simulink model "torqueBalancing"  (Simulink 8.7)
settings: Solver=FixedStepDiscrete  StartTime=0.0  StopTime="CONFIG.SIMULATION_TIME "  FixedStep=CONFIG.Ts  RelTol=1e-3
InitFcn:
  | cd(fileparts(which(bdroot)));
  | initTorqueBalancing;
values from neighbouring files (symbols this model uses):
  baseToWorldRotationPort = ['/' WBT_modelName '/floatingBaseRotationMatrix:i']    [initTorqueBalancing.m]
  WBT_modelName = 'matlabTorqueBalancing'    [initTorqueBalancing.m]
undefined symbols (not defined in the file or in its folder): bVectorConstraints, CONFIG, ConstraintsMatrix, DiscIntNeverNeededParam, gain, references, reg, ROBOT_DOF, ROBOT_DOF_FOR_SIMULINK, sat, SM, sm, WBT_robotName
libraries: WBToolboxLibrary x119, simulink x11
(part 2 of 3)

== system torqueBalancing/DesValues/Internal coordinator/nu ==
  qj : Inport
  w_H_b : Inport  Port=2
  "constraints " : Inport  Port=3
  Get Estimate : WBToolboxLibrary/wholeBodyStates/Get Estimate  estimateType=Joints Velocity  robotName=WBT_robotName  localName=WBT_modelName  wbiFile=WBT_wbiFilename  wbiList=WBT_wbiList
  Jacobian l_sole : WBToolboxLibrary/wholeBodyModel/Jacobians/Jacobian  frameName='l_sole'  robotName=WBT_robotName  localName=WBT_modelName  wbiFile=WBT_wbiFilename  wbiList=WBT_wbiList
  Jacobian r_sole : WBToolboxLibrary/wholeBodyModel/Jacobians/Jacobian  frameName='r_sole'  robotName=WBT_robotName  localName=WBT_modelName  wbiFile=WBT_wbiFilename  wbiList=WBT_wbiList
  MATLAB Function : MATLAB Function  TreatAsAtomicUnit=on
  Mux : Mux  Inputs=2
  vb + Dqj : Outport
  wires:
  Get Estimate/1 -> MATLAB Function/4(qD), Mux/2
  Mux/1 -> vb + Dqj/1
  Jacobian r_sole/1 -> MATLAB Function/2(JcRightFoot)
  "constraints "/1 -> MATLAB Function/3(activeFeetConstraints)
  MATLAB Function/1(y) -> Mux/1
  Jacobian l_sole/1 -> MATLAB Function/1(JcLeftFoot)
  qj/1 -> Jacobian r_sole/2, Jacobian l_sole/2
  w_H_b/1 -> Jacobian r_sole/1, Jacobian l_sole/1

== system torqueBalancing/DesValues/Internal coordinator/refGen ==
  xCom(0) : Inport
  qj(0) : Inport  Port=2
  Enable : EnablePort
  Clock1 : Clock
  refGenFCN : MATLAB Function  TreatAsAtomicUnit=on
  qDes : Outport
  CoMrefs : Outport  Port=2
  wires:
  refGenFCN/2(desired_x_dx_ddx_CoM) -> CoMrefs/1
  xCom(0)/1 -> refGenFCN/1(xCom0)
  Clock1/1 -> refGenFCN/3(t)
  qj(0)/1 -> refGenFCN/2(q0)
  refGenFCN/1(qDes) -> qDes/1

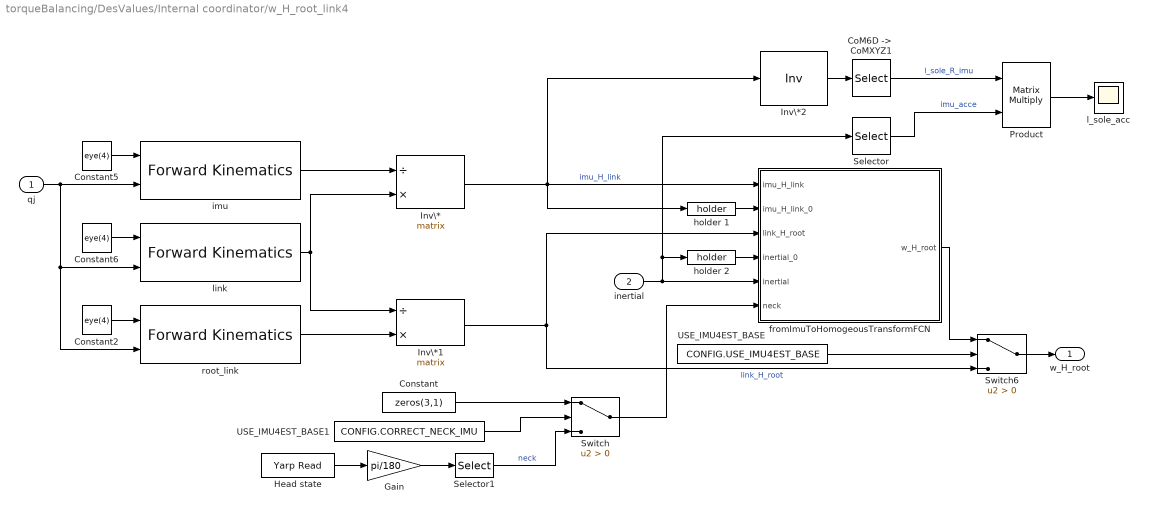
== system torqueBalancing/DesValues/Internal coordinator/w_H_root_link4 ==
  qj : Inport
  inertial : Inport  Port=2
  "CoM6D ->  CoMXYZ1" : Selector  NumberOfDimensions=2  InputPortWidth=7  IndexOptions=Index vector (dialog),Index vector (dialog)  Indices=[1 2 3],[1 2 3]  OutputSizes=1,1
  Constant : Constant  Value=zeros(3,1)
  Constant2 : Constant  Value=eye(4)
  Constant5 : Constant  Value=eye(4)
  Constant6 : Constant  Value=eye(4)
  Gain : Gain  Gain=pi/180
  Head state : WBToolboxLibrary/Utilities/Yarp Read  portName=[WBT_robotName, '/head/state:o']  signalSize=6  blocking=off  timestamp=off  autoconnect=on  errorOnConnection=off
  Inv\* : Product  Inputs=/*  Multiplication=Matrix(*)
  Inv\*1 : Product  Inputs=/*  Multiplication=Matrix(*)
  Inv\*2 : Product  Inputs=/  Multiplication=Matrix(*)
  Product : Product  Multiplication=Matrix(*)
  Selector : Selector  InputPortWidth=12  IndexOptions=Index vector (dialog)  Indices=[4 5 6 ]  OutputSizes=1
  Selector1 : Selector  InputPortWidth=6  IndexOptions=Index vector (dialog)  Indices=[1:3]  OutputSizes=1
  Switch : Switch  Criteria=u2 > Threshold
  Switch6 : Switch  Criteria=u2 > Threshold
  USE_IMU4EST_BASE : Constant  Value=CONFIG.USE_IMU4EST_BASE
  USE_IMU4EST_BASE1 : Constant  Value=CONFIG.CORRECT_NECK_IMU
  fromImuToHomogeousTransformFCN : MATLAB Function  TreatAsAtomicUnit=on
  holder 1 : WBToolboxLibrary/Utilities/holder 
  holder 2 : WBToolboxLibrary/Utilities/holder 
  imu : WBToolboxLibrary/wholeBodyModel/Kinematics/Forward Kinematics  frameName=imu_link_name  robotName=WBT_robotName  localName=WBT_modelName  wbiFile=WBT_wbiFilename  wbiList=WBT_wbiList
  l_sole_acc : Scope
  link : WBToolboxLibrary/wholeBodyModel/Kinematics/Forward Kinematics  frameName=link_name  robotName=WBT_robotName  localName=WBT_modelName  wbiFile=WBT_wbiFilename  wbiList=WBT_wbiList
  root_link : WBToolboxLibrary/wholeBodyModel/Kinematics/Forward Kinematics  frameName=root_link_name  robotName=WBT_robotName  localName=WBT_modelName  wbiFile=WBT_wbiFilename  wbiList=WBT_wbiList
  w_H_root : Outport
  wires:
  Constant5/1 -> imu/1
  Inv\*/1 -> Inv\*2/1, holder 1/1, fromImuToHomogeousTransformFCN/1(imu_H_link)  "imu_H_link"
  imu/1 -> Inv\*/1
  Constant6/1 -> link/1
  Inv\*1/1 -> Switch6/3, fromImuToHomogeousTransformFCN/3(link_H_root)  "link_H_root"
  link/1 -> Inv\*/2, Inv\*1/1
  inertial/1 -> Selector/1, holder 2/1, fromImuToHomogeousTransformFCN/5(inertial)
  Switch6/1 -> w_H_root/1
  USE_IMU4EST_BASE/1 -> Switch6/2
  fromImuToHomogeousTransformFCN/1(w_H_root) -> Switch6/1
  Constant2/1 -> root_link/1
  qj/1 -> root_link/2, link/2, imu/2
  root_link/1 -> Inv\*1/2
  holder 1/1 -> fromImuToHomogeousTransformFCN/2(imu_H_link_0)
  holder 2/1 -> fromImuToHomogeousTransformFCN/4(inertial_0)
  Inv\*2/1 -> "CoM6D ->  CoMXYZ1"/1
  "CoM6D ->  CoMXYZ1"/1 -> Product/1  "l_sole_R_imu"
  Selector/1 -> Product/2  "imu_acce"
  Product/1 -> l_sole_acc/1
  Head state/1 -> Gain/1
  Selector1/1 -> Switch/3  "neck"
  Constant/1 -> Switch/1
  USE_IMU4EST_BASE1/1 -> Switch/2
  Switch/1 -> fromImuToHomogeousTransformFCN/6(neck)
  Gain/1 -> Selector1/1

== system torqueBalancing/DesValues/Internal coordinator/xCom ==
  w_H_b : Inport
  qj : Inport  Port=2
  "CoM6D ->  CoMXYZ2" : Selector  NumberOfDimensions=2  InputPortWidth=7  IndexOptions=Index vector (dialog),Index vector (dialog)  Indices=[1 2 3],[4]  OutputSizes=1,1
  com : WBToolboxLibrary/wholeBodyModel/Kinematics/Forward Kinematics  frameName='com'  robotName=WBT_robotName  localName=WBT_modelName  wbiFile=WBT_wbiFilename  wbiList=WBT_wbiList
  xCom : Outport
  wires:
  qj/1 -> com/2
  "CoM6D ->  CoMXYZ2"/1 -> xCom/1
  com/1 -> "CoM6D ->  CoMXYZ2"/1
  w_H_b/1 -> com/1

== system torqueBalancing/DesValues/State Machine/Visualise extrnal wrenches   ==
  wL_WBDT : Inport
  wR_WBDT : Inport  Port=2
  Enable : EnablePort
  Constant : Constant  Value=sm.wrench.thresholdContactOn
  Constant2 : Constant  Value=sm.wrench.thresholdContactOff
  left foot ext wrench : Scope  NumInputPorts=3
  right foot ext wrench : Scope  NumInputPorts=3
  wires:
  Constant/1 -> left foot ext wrench/2, right foot ext wrench/2  "thresholdContactOn"
  wR_WBDT/1 -> right foot ext wrench/1  "wR_WBDT"
  wL_WBDT/1 -> left foot ext wrench/1  "wL_WBDT"
  Constant2/1 -> left foot ext wrench/3, right foot ext wrench/3  "thresholdContactOff"

== system torqueBalancing/DesValues/State Machine/nu ==
  qj : Inport
  w_H_b : Inport  Port=2
  "constraints " : Inport  Port=3
  Get Estimate : WBToolboxLibrary/wholeBodyStates/Get Estimate  estimateType=Joints Velocity  robotName=WBT_robotName  localName=WBT_modelName  wbiFile=WBT_wbiFilename  wbiList=WBT_wbiList
  Jacobian l_sole : WBToolboxLibrary/wholeBodyModel/Jacobians/Jacobian  frameName='l_sole'  robotName=WBT_robotName  localName=WBT_modelName  wbiFile=WBT_wbiFilename  wbiList=WBT_wbiList
  Jacobian r_sole : WBToolboxLibrary/wholeBodyModel/Jacobians/Jacobian  frameName='r_sole'  robotName=WBT_robotName  localName=WBT_modelName  wbiFile=WBT_wbiFilename  wbiList=WBT_wbiList
  MATLAB Function : MATLAB Function  TreatAsAtomicUnit=on
  Mux : Mux  Inputs=2
  vb + Dqj : Outport
  wires:
  Get Estimate/1 -> MATLAB Function/4(qD), Mux/2
  Mux/1 -> vb + Dqj/1
  Jacobian r_sole/1 -> MATLAB Function/2(JcRightFoot)
  "constraints "/1 -> MATLAB Function/3(activeFeetConstraints)
  MATLAB Function/1(y) -> Mux/1
  Jacobian l_sole/1 -> MATLAB Function/1(JcLeftFoot)
  qj/1 -> Jacobian r_sole/2, Jacobian l_sole/2
  w_H_b/1 -> Jacobian r_sole/1, Jacobian l_sole/1

== system torqueBalancing/DesValues/State Machine/visualise inertial ==
  jointAngles : Inport
  inertial : Inport  Port=2
  Enable : EnablePort
  Inv\* : Product  Inputs=/*  Multiplication=Matrix(*)
  Inv\*1 : Product  Inputs=/*  Multiplication=Matrix(*)
  Visualize hom transf1 : Subsystem
  Visualize hom transf2 : Subsystem
  Visualize hom transf3 : Subsystem
  Visualize hom transf4 : Subsystem
  Visualize hom transf5 : Subsystem
  Visualize hom transf6 : Subsystem
  "inertial -> rpy" : Selector  InputPortWidth=12  IndexOptions=Index vector (dialog)  Indices=[1 2 3]  OutputSizes=1
  l_sole_H_root_link2 : Subsystem  mask{link_name='l_sole'}
  l_sole_H_root_link3 : Subsystem  mask{link_name='r_sole'}
  rpy : Scope
  w_H_root_link1 : Subsystem  mask{link_name='r_sole'}
      mask prompts: link_name "link name"
      mask help:
      | This block evaluates the homogeneous transformation between the world and the root link, i.e. ^wH_b. It assumes that the link specified by the variable 'link_name' has a constant position
      | w.r.t. an inertial frame, but it can rotate arbitrarily. This rotation is retrived from the IMU sensor.
      mask Display:
      | str = strrep(link_name, '_','\_');
      | port_label('output',1,['{}^{',str '}H_{root}'],'texmode','on')
      | clear str;
      | 
      | port_label('input',1,'q_j','texmode','on')
      | 
      | port_label('input',2,'inertial','texmode','on')
  w_H_root_link4 : Subsystem  mask{link_name='l_sole'}
      mask prompts: link_name "link name"
      mask help:
      | This block evaluates the homogeneous transformation between the world and the root link, i.e. ^wH_b. It assumes that the link specified by the variable 'link_name' has a constant position
      | w.r.t. an inertial frame, but it can rotate arbitrarily. This rotation is retrived from the IMU sensor.
      mask Display:
      | str = strrep(link_name, '_','\_');
      | port_label('output',1,['{}^{',str '}H_{root}'],'texmode','on')
      | clear str;
      | 
      | port_label('input',1,'q_j','texmode','on')
      | 
      | port_label('input',2,'inertial','texmode','on')
  wires:
  inertial/1 -> "inertial -> rpy"/1, w_H_root_link1/2(inertial), w_H_root_link4/2(inertial)
  jointAngles/1 -> l_sole_H_root_link2/1(qj), w_H_root_link4/1(qj), w_H_root_link1/1(qj), l_sole_H_root_link3/1(qj)
  l_sole_H_root_link2/1(link_name_H_root_link) -> Visualize hom transf6/1(H), Inv\*/1  "l_sole_H_root_link"
  Inv\*/1 -> Visualize hom transf5/1(H)
  w_H_root_link4/1(w_H_root) -> Visualize hom transf4/1(H), Inv\*/2
  "inertial -> rpy"/1 -> rpy/1
  l_sole_H_root_link3/1(link_name_H_root_link) -> Visualize hom transf2/1(H), Inv\*1/1  "r_sole_H_root_link"
  Inv\*1/1 -> Visualize hom transf1/1(H)
  w_H_root_link1/1(w_H_root) -> Visualize hom transf3/1(H), Inv\*1/2

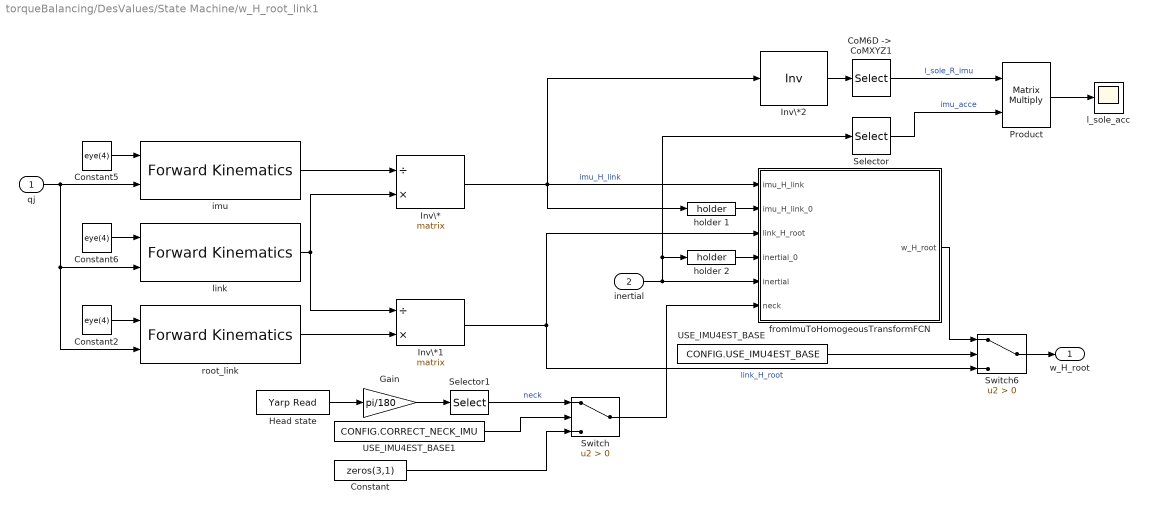
== system torqueBalancing/DesValues/State Machine/w_H_root_link1 ==
  qj : Inport
  inertial : Inport  Port=2
  "CoM6D ->  CoMXYZ1" : Selector  NumberOfDimensions=2  InputPortWidth=7  IndexOptions=Index vector (dialog),Index vector (dialog)  Indices=[1 2 3],[1 2 3]  OutputSizes=1,1
  Constant : Constant  Value=zeros(3,1)
  Constant2 : Constant  Value=eye(4)
  Constant5 : Constant  Value=eye(4)
  Constant6 : Constant  Value=eye(4)
  Gain : Gain  Gain=pi/180
  Head state : WBToolboxLibrary/Utilities/Yarp Read  portName=[WBT_robotName, '/head/state:o']  signalSize=6  blocking=off  timestamp=off  autoconnect=on  errorOnConnection=off
  Inv\* : Product  Inputs=/*  Multiplication=Matrix(*)
  Inv\*1 : Product  Inputs=/*  Multiplication=Matrix(*)
  Inv\*2 : Product  Inputs=/  Multiplication=Matrix(*)
  Product : Product  Multiplication=Matrix(*)
  Selector : Selector  InputPortWidth=12  IndexOptions=Index vector (dialog)  Indices=[4 5 6 ]  OutputSizes=1
  Selector1 : Selector  InputPortWidth=6  IndexOptions=Index vector (dialog)  Indices=[1:3]  OutputSizes=1
  Switch : Switch  Criteria=u2 > Threshold
  Switch6 : Switch  Criteria=u2 > Threshold
  USE_IMU4EST_BASE : Constant  Value=CONFIG.USE_IMU4EST_BASE
  USE_IMU4EST_BASE1 : Constant  Value=CONFIG.CORRECT_NECK_IMU
  fromImuToHomogeousTransformFCN : MATLAB Function  TreatAsAtomicUnit=on
  holder 1 : WBToolboxLibrary/Utilities/holder 
  holder 2 : WBToolboxLibrary/Utilities/holder 
  imu : WBToolboxLibrary/wholeBodyModel/Kinematics/Forward Kinematics  frameName=imu_link_name  robotName=WBT_robotName  localName=WBT_modelName  wbiFile=WBT_wbiFilename  wbiList=WBT_wbiList
  l_sole_acc : Scope
  link : WBToolboxLibrary/wholeBodyModel/Kinematics/Forward Kinematics  frameName=link_name  robotName=WBT_robotName  localName=WBT_modelName  wbiFile=WBT_wbiFilename  wbiList=WBT_wbiList
  root_link : WBToolboxLibrary/wholeBodyModel/Kinematics/Forward Kinematics  frameName=root_link_name  robotName=WBT_robotName  localName=WBT_modelName  wbiFile=WBT_wbiFilename  wbiList=WBT_wbiList
  w_H_root : Outport
  wires:
  Constant5/1 -> imu/1
  Inv\*/1 -> Inv\*2/1, holder 1/1, fromImuToHomogeousTransformFCN/1(imu_H_link)  "imu_H_link"
  imu/1 -> Inv\*/1
  Constant6/1 -> link/1
  Inv\*1/1 -> Switch6/3, fromImuToHomogeousTransformFCN/3(link_H_root)  "link_H_root"
  link/1 -> Inv\*/2, Inv\*1/1
  inertial/1 -> Selector/1, holder 2/1, fromImuToHomogeousTransformFCN/5(inertial)
  Switch6/1 -> w_H_root/1
  USE_IMU4EST_BASE/1 -> Switch6/2
  fromImuToHomogeousTransformFCN/1(w_H_root) -> Switch6/1
  Constant2/1 -> root_link/1
  qj/1 -> root_link/2, link/2, imu/2
  root_link/1 -> Inv\*1/2
  holder 1/1 -> fromImuToHomogeousTransformFCN/2(imu_H_link_0)
  holder 2/1 -> fromImuToHomogeousTransformFCN/4(inertial_0)
  Inv\*2/1 -> "CoM6D ->  CoMXYZ1"/1
  "CoM6D ->  CoMXYZ1"/1 -> Product/1  "l_sole_R_imu"
  Selector/1 -> Product/2  "imu_acce"
  Product/1 -> l_sole_acc/1
  Head state/1 -> Gain/1
  Selector1/1 -> Switch/1  "neck"
  USE_IMU4EST_BASE1/1 -> Switch/2
  Switch/1 -> fromImuToHomogeousTransformFCN/6(neck)
  Gain/1 -> Selector1/1
  Constant/1 -> Switch/3

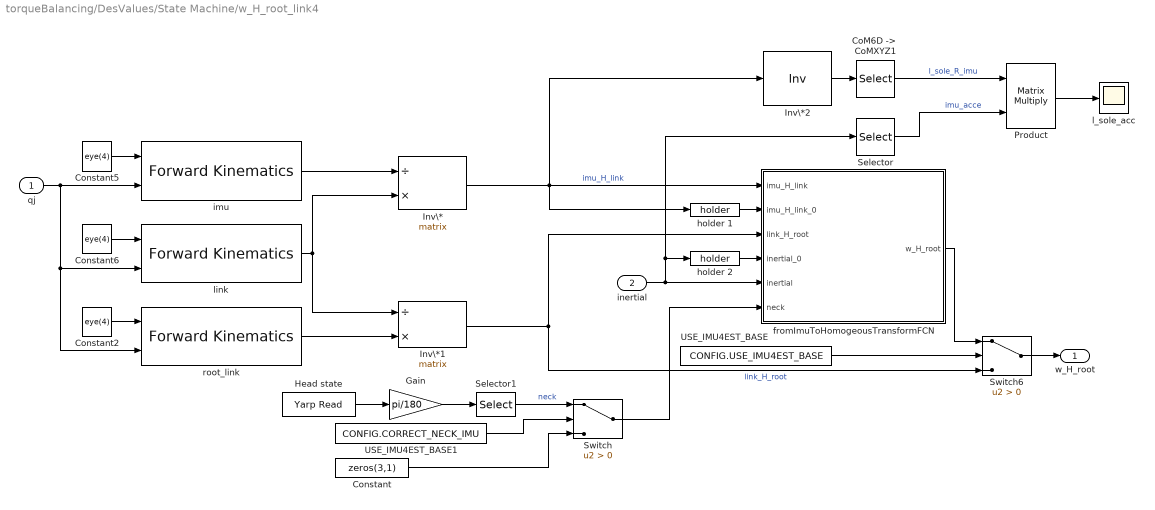
== system torqueBalancing/DesValues/State Machine/w_H_root_link4 ==
  qj : Inport
  inertial : Inport  Port=2
  "CoM6D ->  CoMXYZ1" : Selector  NumberOfDimensions=2  InputPortWidth=7  IndexOptions=Index vector (dialog),Index vector (dialog)  Indices=[1 2 3],[1 2 3]  OutputSizes=1,1
  Constant : Constant  Value=zeros(3,1)
  Constant2 : Constant  Value=eye(4)
  Constant5 : Constant  Value=eye(4)
  Constant6 : Constant  Value=eye(4)
  Gain : Gain  Gain=pi/180
  Head state : WBToolboxLibrary/Utilities/Yarp Read  portName=[WBT_robotName, '/head/state:o']  signalSize=6  blocking=off  timestamp=off  autoconnect=on  errorOnConnection=off
  Inv\* : Product  Inputs=/*  Multiplication=Matrix(*)
  Inv\*1 : Product  Inputs=/*  Multiplication=Matrix(*)
  Inv\*2 : Product  Inputs=/  Multiplication=Matrix(*)
  Product : Product  Multiplication=Matrix(*)
  Selector : Selector  InputPortWidth=12  IndexOptions=Index vector (dialog)  Indices=[4 5 6 ]  OutputSizes=1
  Selector1 : Selector  InputPortWidth=6  IndexOptions=Index vector (dialog)  Indices=[1:3]  OutputSizes=1
  Switch : Switch  Criteria=u2 > Threshold
  Switch6 : Switch  Criteria=u2 > Threshold
  USE_IMU4EST_BASE : Constant  Value=CONFIG.USE_IMU4EST_BASE
  USE_IMU4EST_BASE1 : Constant  Value=CONFIG.CORRECT_NECK_IMU
  fromImuToHomogeousTransformFCN : MATLAB Function  TreatAsAtomicUnit=on
  holder 1 : WBToolboxLibrary/Utilities/holder 
  holder 2 : WBToolboxLibrary/Utilities/holder 
  imu : WBToolboxLibrary/wholeBodyModel/Kinematics/Forward Kinematics  frameName=imu_link_name  robotName=WBT_robotName  localName=WBT_modelName  wbiFile=WBT_wbiFilename  wbiList=WBT_wbiList
  l_sole_acc : Scope
  link : WBToolboxLibrary/wholeBodyModel/Kinematics/Forward Kinematics  frameName=link_name  robotName=WBT_robotName  localName=WBT_modelName  wbiFile=WBT_wbiFilename  wbiList=WBT_wbiList
  root_link : WBToolboxLibrary/wholeBodyModel/Kinematics/Forward Kinematics  frameName=root_link_name  robotName=WBT_robotName  localName=WBT_modelName  wbiFile=WBT_wbiFilename  wbiList=WBT_wbiList
  w_H_root : Outport
  wires:
  Constant5/1 -> imu/1
  Inv\*/1 -> Inv\*2/1, holder 1/1, fromImuToHomogeousTransformFCN/1(imu_H_link)  "imu_H_link"
  imu/1 -> Inv\*/1
  Constant6/1 -> link/1
  Inv\*1/1 -> Switch6/3, fromImuToHomogeousTransformFCN/3(link_H_root)  "link_H_root"
  link/1 -> Inv\*/2, Inv\*1/1
  inertial/1 -> Selector/1, holder 2/1, fromImuToHomogeousTransformFCN/5(inertial)
  Switch6/1 -> w_H_root/1
  USE_IMU4EST_BASE/1 -> Switch6/2
  fromImuToHomogeousTransformFCN/1(w_H_root) -> Switch6/1
  Constant2/1 -> root_link/1
  qj/1 -> root_link/2, link/2, imu/2
  root_link/1 -> Inv\*1/2
  holder 1/1 -> fromImuToHomogeousTransformFCN/2(imu_H_link_0)
  holder 2/1 -> fromImuToHomogeousTransformFCN/4(inertial_0)
  Inv\*2/1 -> "CoM6D ->  CoMXYZ1"/1
  "CoM6D ->  CoMXYZ1"/1 -> Product/1  "l_sole_R_imu"
  Selector/1 -> Product/2  "imu_acce"
  Product/1 -> l_sole_acc/1
  Head state/1 -> Gain/1
  Selector1/1 -> Switch/1  "neck"
  USE_IMU4EST_BASE1/1 -> Switch/2
  Switch/1 -> fromImuToHomogeousTransformFCN/6(neck)
  Gain/1 -> Selector1/1
  Constant/1 -> Switch/3

== system torqueBalancing/DesValues/State Machine/xCom ==
  qj : Inport
  w_H_b : Inport  Port=2
  "CoM6D ->  CoMXYZ2" : Selector  NumberOfDimensions=2  InputPortWidth=7  IndexOptions=Index vector (dialog),Index vector (dialog)  Indices=[1 2 3],[4]  OutputSizes=1,1
  com : WBToolboxLibrary/wholeBodyModel/Kinematics/Forward Kinematics  frameName='com'  robotName=WBT_robotName  localName=WBT_modelName  wbiFile=WBT_wbiFilename  wbiList=WBT_wbiList
  xCom : Outport
  wires:
  qj/1 -> com/2
  "CoM6D ->  CoMXYZ2"/1 -> xCom/1
  com/1 -> "CoM6D ->  CoMXYZ2"/1
  w_H_b/1 -> com/1

== system torqueBalancing/DesValues/State Machine/xCom1 ==
  qj : Inport
  w_H_b : Inport  Port=2
  "CoM6D ->  CoMXYZ2" : Selector  NumberOfDimensions=2  InputPortWidth=7  IndexOptions=Index vector (dialog),Index vector (dialog)  Indices=[1 2 3],[4]  OutputSizes=1,1
  com : WBToolboxLibrary/wholeBodyModel/Kinematics/Forward Kinematics  frameName='com'  robotName=WBT_robotName  localName=WBT_modelName  wbiFile=WBT_wbiFilename  wbiList=WBT_wbiList
  xCom : Outport
  wires:
  qj/1 -> com/2
  "CoM6D ->  CoMXYZ2"/1 -> xCom/1
  com/1 -> "CoM6D ->  CoMXYZ2"/1
  w_H_b/1 -> com/1

== system torqueBalancing/DesValues/State Machine Walking/Visualise extrnal wrenches   ==
  wL_WBDT : Inport
  wR_WBDT : Inport  Port=2
  Enable : EnablePort
  left foot ext wrench : Scope
  right foot ext wrench : Scope
  wires:
  wR_WBDT/1 -> right foot ext wrench/1  "wR_WBDT"
  wL_WBDT/1 -> left foot ext wrench/1  "wL_WBDT"

== system torqueBalancing/DesValues/State Machine Walking/nu ==
  qj : Inport
  w_H_b : Inport  Port=2
  "constraints " : Inport  Port=3
  Get Estimate : WBToolboxLibrary/wholeBodyStates/Get Estimate  estimateType=Joints Velocity  robotName=WBT_robotName  localName=WBT_modelName  wbiFile=WBT_wbiFilename  wbiList=WBT_wbiList
  Jacobian l_sole : WBToolboxLibrary/wholeBodyModel/Jacobians/Jacobian  frameName='l_sole'  robotName=WBT_robotName  localName=WBT_modelName  wbiFile=WBT_wbiFilename  wbiList=WBT_wbiList
  Jacobian r_sole : WBToolboxLibrary/wholeBodyModel/Jacobians/Jacobian  frameName='r_sole'  robotName=WBT_robotName  localName=WBT_modelName  wbiFile=WBT_wbiFilename  wbiList=WBT_wbiList
  MATLAB Function : MATLAB Function  TreatAsAtomicUnit=on
  Mux : Mux  Inputs=2
  vb + Dqj : Outport
  wires:
  Get Estimate/1 -> MATLAB Function/4(qD), Mux/2
  Mux/1 -> vb + Dqj/1
  Jacobian r_sole/1 -> MATLAB Function/2(JcRightFoot)
  "constraints "/1 -> MATLAB Function/3(activeFeetConstraints)
  MATLAB Function/1(y) -> Mux/1
  Jacobian l_sole/1 -> MATLAB Function/1(JcLeftFoot)
  qj/1 -> Jacobian r_sole/2, Jacobian l_sole/2
  w_H_b/1 -> Jacobian r_sole/1, Jacobian l_sole/1

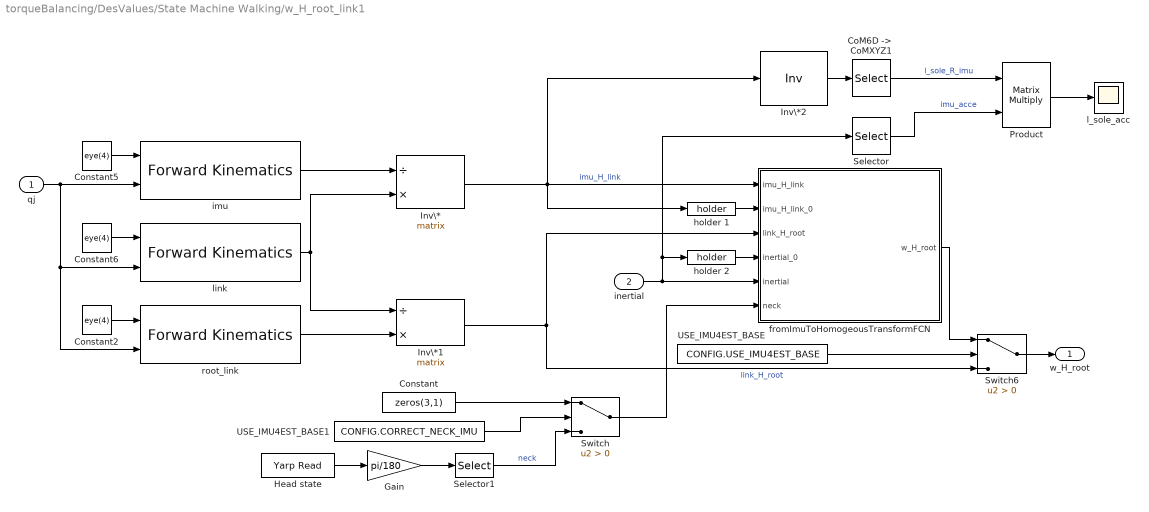
== system torqueBalancing/DesValues/State Machine Walking/w_H_root_link1 ==
  qj : Inport
  inertial : Inport  Port=2
  "CoM6D ->  CoMXYZ1" : Selector  NumberOfDimensions=2  InputPortWidth=7  IndexOptions=Index vector (dialog),Index vector (dialog)  Indices=[1 2 3],[1 2 3]  OutputSizes=1,1
  Constant : Constant  Value=zeros(3,1)
  Constant2 : Constant  Value=eye(4)
  Constant5 : Constant  Value=eye(4)
  Constant6 : Constant  Value=eye(4)
  Gain : Gain  Gain=pi/180
  Head state : WBToolboxLibrary/Utilities/Yarp Read  portName=[WBT_robotName, '/head/state:o']  signalSize=6  blocking=off  timestamp=off  autoconnect=on  errorOnConnection=off
  Inv\* : Product  Inputs=/*  Multiplication=Matrix(*)
  Inv\*1 : Product  Inputs=/*  Multiplication=Matrix(*)
  Inv\*2 : Product  Inputs=/  Multiplication=Matrix(*)
  Product : Product  Multiplication=Matrix(*)
  Selector : Selector  InputPortWidth=12  IndexOptions=Index vector (dialog)  Indices=[4 5 6 ]  OutputSizes=1
  Selector1 : Selector  InputPortWidth=6  IndexOptions=Index vector (dialog)  Indices=[1:3]  OutputSizes=1
  Switch : Switch  Criteria=u2 > Threshold
  Switch6 : Switch  Criteria=u2 > Threshold
  USE_IMU4EST_BASE : Constant  Value=CONFIG.USE_IMU4EST_BASE
  USE_IMU4EST_BASE1 : Constant  Value=CONFIG.CORRECT_NECK_IMU
  fromImuToHomogeousTransformFCN : MATLAB Function  TreatAsAtomicUnit=on
  holder 1 : WBToolboxLibrary/Utilities/holder 
  holder 2 : WBToolboxLibrary/Utilities/holder 
  imu : WBToolboxLibrary/wholeBodyModel/Kinematics/Forward Kinematics  frameName=imu_link_name  robotName=WBT_robotName  localName=WBT_modelName  wbiFile=WBT_wbiFilename  wbiList=WBT_wbiList
  l_sole_acc : Scope
  link : WBToolboxLibrary/wholeBodyModel/Kinematics/Forward Kinematics  frameName=link_name  robotName=WBT_robotName  localName=WBT_modelName  wbiFile=WBT_wbiFilename  wbiList=WBT_wbiList
  root_link : WBToolboxLibrary/wholeBodyModel/Kinematics/Forward Kinematics  frameName=root_link_name  robotName=WBT_robotName  localName=WBT_modelName  wbiFile=WBT_wbiFilename  wbiList=WBT_wbiList
  w_H_root : Outport
  wires:
  Constant5/1 -> imu/1
  Inv\*/1 -> Inv\*2/1, holder 1/1, fromImuToHomogeousTransformFCN/1(imu_H_link)  "imu_H_link"
  imu/1 -> Inv\*/1
  Constant6/1 -> link/1
  Inv\*1/1 -> Switch6/3, fromImuToHomogeousTransformFCN/3(link_H_root)  "link_H_root"
  link/1 -> Inv\*/2, Inv\*1/1
  inertial/1 -> Selector/1, holder 2/1, fromImuToHomogeousTransformFCN/5(inertial)
  Switch6/1 -> w_H_root/1
  USE_IMU4EST_BASE/1 -> Switch6/2
  fromImuToHomogeousTransformFCN/1(w_H_root) -> Switch6/1
  Constant2/1 -> root_link/1
  qj/1 -> root_link/2, link/2, imu/2
  root_link/1 -> Inv\*1/2
  holder 1/1 -> fromImuToHomogeousTransformFCN/2(imu_H_link_0)
  holder 2/1 -> fromImuToHomogeousTransformFCN/4(inertial_0)
  Inv\*2/1 -> "CoM6D ->  CoMXYZ1"/1
  "CoM6D ->  CoMXYZ1"/1 -> Product/1  "l_sole_R_imu"
  Selector/1 -> Product/2  "imu_acce"
  Product/1 -> l_sole_acc/1
  Head state/1 -> Gain/1
  Selector1/1 -> Switch/3  "neck"
  Constant/1 -> Switch/1
  USE_IMU4EST_BASE1/1 -> Switch/2
  Switch/1 -> fromImuToHomogeousTransformFCN/6(neck)
  Gain/1 -> Selector1/1

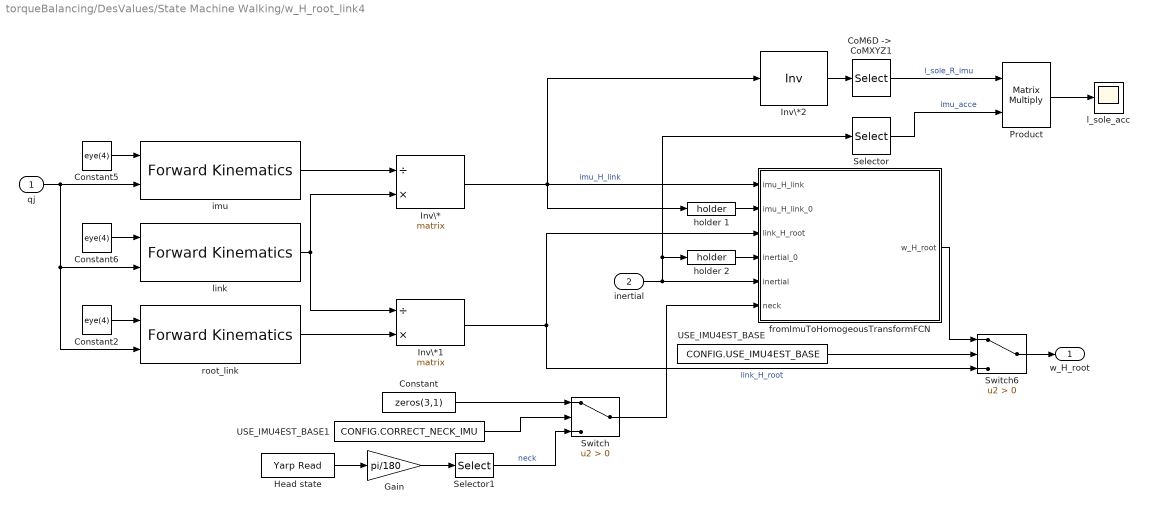
== system torqueBalancing/DesValues/State Machine Walking/w_H_root_link4 ==
  qj : Inport
  inertial : Inport  Port=2
  "CoM6D ->  CoMXYZ1" : Selector  NumberOfDimensions=2  InputPortWidth=7  IndexOptions=Index vector (dialog),Index vector (dialog)  Indices=[1 2 3],[1 2 3]  OutputSizes=1,1
  Constant : Constant  Value=zeros(3,1)
  Constant2 : Constant  Value=eye(4)
  Constant5 : Constant  Value=eye(4)
  Constant6 : Constant  Value=eye(4)
  Gain : Gain  Gain=pi/180
  Head state : WBToolboxLibrary/Utilities/Yarp Read  portName=[WBT_robotName, '/head/state:o']  signalSize=6  blocking=off  timestamp=off  autoconnect=on  errorOnConnection=off
  Inv\* : Product  Inputs=/*  Multiplication=Matrix(*)
  Inv\*1 : Product  Inputs=/*  Multiplication=Matrix(*)
  Inv\*2 : Product  Inputs=/  Multiplication=Matrix(*)
  Product : Product  Multiplication=Matrix(*)
  Selector : Selector  InputPortWidth=12  IndexOptions=Index vector (dialog)  Indices=[4 5 6 ]  OutputSizes=1
  Selector1 : Selector  InputPortWidth=6  IndexOptions=Index vector (dialog)  Indices=[1:3]  OutputSizes=1
  Switch : Switch  Criteria=u2 > Threshold
  Switch6 : Switch  Criteria=u2 > Threshold
  USE_IMU4EST_BASE : Constant  Value=CONFIG.USE_IMU4EST_BASE
  USE_IMU4EST_BASE1 : Constant  Value=CONFIG.CORRECT_NECK_IMU
  fromImuToHomogeousTransformFCN : MATLAB Function  TreatAsAtomicUnit=on
  holder 1 : WBToolboxLibrary/Utilities/holder 
  holder 2 : WBToolboxLibrary/Utilities/holder 
  imu : WBToolboxLibrary/wholeBodyModel/Kinematics/Forward Kinematics  frameName=imu_link_name  robotName=WBT_robotName  localName=WBT_modelName  wbiFile=WBT_wbiFilename  wbiList=WBT_wbiList
  l_sole_acc : Scope
  link : WBToolboxLibrary/wholeBodyModel/Kinematics/Forward Kinematics  frameName=link_name  robotName=WBT_robotName  localName=WBT_modelName  wbiFile=WBT_wbiFilename  wbiList=WBT_wbiList
  root_link : WBToolboxLibrary/wholeBodyModel/Kinematics/Forward Kinematics  frameName=root_link_name  robotName=WBT_robotName  localName=WBT_modelName  wbiFile=WBT_wbiFilename  wbiList=WBT_wbiList
  w_H_root : Outport
  wires:
  Constant5/1 -> imu/1
  Inv\*/1 -> Inv\*2/1, holder 1/1, fromImuToHomogeousTransformFCN/1(imu_H_link)  "imu_H_link"
  imu/1 -> Inv\*/1
  Constant6/1 -> link/1
  Inv\*1/1 -> Switch6/3, fromImuToHomogeousTransformFCN/3(link_H_root)  "link_H_root"
  link/1 -> Inv\*/2, Inv\*1/1
  inertial/1 -> Selector/1, holder 2/1, fromImuToHomogeousTransformFCN/5(inertial)
  Switch6/1 -> w_H_root/1
  USE_IMU4EST_BASE/1 -> Switch6/2
  fromImuToHomogeousTransformFCN/1(w_H_root) -> Switch6/1
  Constant2/1 -> root_link/1
  qj/1 -> root_link/2, link/2, imu/2
  root_link/1 -> Inv\*1/2
  holder 1/1 -> fromImuToHomogeousTransformFCN/2(imu_H_link_0)
  holder 2/1 -> fromImuToHomogeousTransformFCN/4(inertial_0)
  Inv\*2/1 -> "CoM6D ->  CoMXYZ1"/1
  "CoM6D ->  CoMXYZ1"/1 -> Product/1  "l_sole_R_imu"
  Selector/1 -> Product/2  "imu_acce"
  Product/1 -> l_sole_acc/1
  Head state/1 -> Gain/1
  Selector1/1 -> Switch/3  "neck"
  Constant/1 -> Switch/1
  USE_IMU4EST_BASE1/1 -> Switch/2
  Switch/1 -> fromImuToHomogeousTransformFCN/6(neck)
  Gain/1 -> Selector1/1

== system torqueBalancing/DesValues/State Machine Walking/xCom ==
  qj : Inport
  w_H_b : Inport  Port=2
  "CoM6D ->  CoMXYZ2" : Selector  NumberOfDimensions=2  InputPortWidth=7  IndexOptions=Index vector (dialog),Index vector (dialog)  Indices=[1 2 3],[4]  OutputSizes=1,1
  com : WBToolboxLibrary/wholeBodyModel/Kinematics/Forward Kinematics  frameName='com'  robotName=WBT_robotName  localName=WBT_modelName  wbiFile=WBT_wbiFilename  wbiList=WBT_wbiList
  xCom : Outport
  wires:
  qj/1 -> com/2
  "CoM6D ->  CoMXYZ2"/1 -> xCom/1
  com/1 -> "CoM6D ->  CoMXYZ2"/1
  w_H_b/1 -> com/1

== system torqueBalancing/DesValues/State Machine Walking/xCom1 ==
  qj : Inport
  w_H_b : Inport  Port=2
  "CoM6D ->  CoMXYZ2" : Selector  NumberOfDimensions=2  InputPortWidth=7  IndexOptions=Index vector (dialog),Index vector (dialog)  Indices=[1 2 3],[4]  OutputSizes=1,1
  com : WBToolboxLibrary/wholeBodyModel/Kinematics/Forward Kinematics  frameName='com'  robotName=WBT_robotName  localName=WBT_modelName  wbiFile=WBT_wbiFilename  wbiList=WBT_wbiList
  xCom : Outport
  wires:
  qj/1 -> com/2
  "CoM6D ->  CoMXYZ2"/1 -> xCom/1
  com/1 -> "CoM6D ->  CoMXYZ2"/1
  w_H_b/1 -> com/1

== system torqueBalancing/controller_QP/QP/Visualize eventual QP failures ==
  exitFlagQP : Inport
  state : Inport  Port=2
  Enable : EnablePort
  "QP status (0: no failure, 1: not using)" : Scope  NumInputPorts=2
  wires:
  exitFlagQP/1 -> "QP status (0: no failure, 1: not using)"/1  "exitFlagQP"
  state/1 -> "QP status (0: no failure, 1: not using)"/2

== system torqueBalancing/controller_QP/integralOf Hw1/w_H_root_link4 ==
  qj : Inport
  inertial : Inport  Port=2
  "CoM6D ->  CoMXYZ1" : Selector  NumberOfDimensions=2  InputPortWidth=7  IndexOptions=Index vector (dialog),Index vector (dialog)  Indices=[1 2 3],[1 2 3]  OutputSizes=1,1
  Constant : Constant  Value=zeros(3,1)
  Constant2 : Constant  Value=eye(4)
  Constant5 : Constant  Value=eye(4)
  Constant6 : Constant  Value=eye(4)
  Gain : Gain  Gain=pi/180
  Head state : WBToolboxLibrary/Utilities/Yarp Read  portName=[WBT_robotName, '/head/state:o']  signalSize=6  blocking=off  timestamp=off  autoconnect=on  errorOnConnection=off
  Inv\* : Product  Inputs=/*  Multiplication=Matrix(*)
  Inv\*1 : Product  Inputs=/*  Multiplication=Matrix(*)
  Inv\*2 : Product  Inputs=/  Multiplication=Matrix(*)
  Product : Product  Multiplication=Matrix(*)
  Selector : Selector  InputPortWidth=12  IndexOptions=Index vector (dialog)  Indices=[4 5 6 ]  OutputSizes=1
  Selector1 : Selector  InputPortWidth=6  IndexOptions=Index vector (dialog)  Indices=[1:3]  OutputSizes=1
  Switch : Switch  Criteria=u2 > Threshold
  Switch6 : Switch  Criteria=u2 > Threshold
  USE_IMU4EST_BASE : Constant  Value=CONFIG.USE_IMU4EST_BASE
  USE_IMU4EST_BASE1 : Constant  Value=CONFIG.CORRECT_NECK_IMU
  fromImuToHomogeousTransformFCN : MATLAB Function  TreatAsAtomicUnit=on
  holder 1 : WBToolboxLibrary/Utilities/holder 
  holder 2 : WBToolboxLibrary/Utilities/holder 
  imu : WBToolboxLibrary/wholeBodyModel/Kinematics/Forward Kinematics  frameName=imu_link_name  robotName=WBT_robotName  localName=WBT_modelName  wbiFile=WBT_wbiFilename  wbiList=WBT_wbiList
  l_sole_acc : Scope
  link : WBToolboxLibrary/wholeBodyModel/Kinematics/Forward Kinematics  frameName=link_name  robotName=WBT_robotName  localName=WBT_modelName  wbiFile=WBT_wbiFilename  wbiList=WBT_wbiList
  root_link : WBToolboxLibrary/wholeBodyModel/Kinematics/Forward Kinematics  frameName=root_link_name  robotName=WBT_robotName  localName=WBT_modelName  wbiFile=WBT_wbiFilename  wbiList=WBT_wbiList
  w_H_root : Outport
  wires:
  Constant5/1 -> imu/1
  Inv\*/1 -> Inv\*2/1, holder 1/1, fromImuToHomogeousTransformFCN/1(imu_H_link)  "imu_H_link"
  imu/1 -> Inv\*/1
  Constant6/1 -> link/1
  Inv\*1/1 -> Switch6/3, fromImuToHomogeousTransformFCN/3(link_H_root)  "link_H_root"
  link/1 -> Inv\*/2, Inv\*1/1
  inertial/1 -> Selector/1, holder 2/1, fromImuToHomogeousTransformFCN/5(inertial)
  Switch6/1 -> w_H_root/1
  USE_IMU4EST_BASE/1 -> Switch6/2
  fromImuToHomogeousTransformFCN/1(w_H_root) -> Switch6/1
  Constant2/1 -> root_link/1
  qj/1 -> root_link/2, link/2, imu/2
  root_link/1 -> Inv\*1/2
  holder 1/1 -> fromImuToHomogeousTransformFCN/2(imu_H_link_0)
  holder 2/1 -> fromImuToHomogeousTransformFCN/4(inertial_0)
  Inv\*2/1 -> "CoM6D ->  CoMXYZ1"/1
  "CoM6D ->  CoMXYZ1"/1 -> Product/1  "l_sole_R_imu"
  Selector/1 -> Product/2  "imu_acce"
  Product/1 -> l_sole_acc/1
  Head state/1 -> Gain/1
  Selector1/1 -> Switch/3  "neck"
  Constant/1 -> Switch/1
  USE_IMU4EST_BASE1/1 -> Switch/2
  Switch/1 -> fromImuToHomogeousTransformFCN/6(neck)
  Gain/1 -> Selector1/1

== system torqueBalancing/DesValues/State Machine/visualise inertial/Visualize hom transf1 ==
  H : Inport
  "CoM6D ->  CoMXYZ1" : Selector  NumberOfDimensions=2  InputPortWidth=7  IndexOptions=Index vector (dialog),Index vector (dialog)  Indices=[1 2 3],[1 2 3]  OutputSizes=1,1
  "CoM6D ->  CoMXYZ2" : Selector  NumberOfDimensions=2  InputPortWidth=7  IndexOptions=Index vector (dialog),Index vector (dialog)  Indices=[1 2 3],[4]  OutputSizes=1,1
  Hom : Scope
  MATLAB Function : MATLAB Function  TreatAsAtomicUnit=on
  p : Scope
  rollPitchYaw : Scope
  wires:
  "CoM6D ->  CoMXYZ2"/1 -> p/1
  H/1 -> "CoM6D ->  CoMXYZ2"/1, Hom/1, "CoM6D ->  CoMXYZ1"/1
  "CoM6D ->  CoMXYZ1"/1 -> MATLAB Function/1(R)
  MATLAB Function/1(rollPitchYaw) -> rollPitchYaw/1

== system torqueBalancing/DesValues/State Machine/visualise inertial/Visualize hom transf2 ==
  H : Inport
  "CoM6D ->  CoMXYZ1" : Selector  NumberOfDimensions=2  InputPortWidth=7  IndexOptions=Index vector (dialog),Index vector (dialog)  Indices=[1 2 3],[1 2 3]  OutputSizes=1,1
  "CoM6D ->  CoMXYZ2" : Selector  NumberOfDimensions=2  InputPortWidth=7  IndexOptions=Index vector (dialog),Index vector (dialog)  Indices=[1 2 3],[4]  OutputSizes=1,1
  Hom : Scope
  MATLAB Function : MATLAB Function  TreatAsAtomicUnit=on
  p : Scope
  rollPitchYaw : Scope
  wires:
  "CoM6D ->  CoMXYZ2"/1 -> p/1
  H/1 -> "CoM6D ->  CoMXYZ2"/1, Hom/1, "CoM6D ->  CoMXYZ1"/1
  "CoM6D ->  CoMXYZ1"/1 -> MATLAB Function/1(R)
  MATLAB Function/1(rollPitchYaw) -> rollPitchYaw/1

== system torqueBalancing/DesValues/State Machine/visualise inertial/Visualize hom transf3 ==
  H : Inport
  "CoM6D ->  CoMXYZ1" : Selector  NumberOfDimensions=2  InputPortWidth=7  IndexOptions=Index vector (dialog),Index vector (dialog)  Indices=[1 2 3],[1 2 3]  OutputSizes=1,1
  "CoM6D ->  CoMXYZ2" : Selector  NumberOfDimensions=2  InputPortWidth=7  IndexOptions=Index vector (dialog),Index vector (dialog)  Indices=[1 2 3],[4]  OutputSizes=1,1
  Hom : Scope
  MATLAB Function : MATLAB Function  TreatAsAtomicUnit=on
  p : Scope
  rollPitchYaw : Scope
  wires:
  "CoM6D ->  CoMXYZ2"/1 -> p/1
  H/1 -> "CoM6D ->  CoMXYZ2"/1, Hom/1, "CoM6D ->  CoMXYZ1"/1
  "CoM6D ->  CoMXYZ1"/1 -> MATLAB Function/1(R)
  MATLAB Function/1(rollPitchYaw) -> rollPitchYaw/1

== system torqueBalancing/DesValues/State Machine/visualise inertial/Visualize hom transf4 ==
  H : Inport
  "CoM6D ->  CoMXYZ1" : Selector  NumberOfDimensions=2  InputPortWidth=7  IndexOptions=Index vector (dialog),Index vector (dialog)  Indices=[1 2 3],[1 2 3]  OutputSizes=1,1
  "CoM6D ->  CoMXYZ2" : Selector  NumberOfDimensions=2  InputPortWidth=7  IndexOptions=Index vector (dialog),Index vector (dialog)  Indices=[1 2 3],[4]  OutputSizes=1,1
  Hom : Scope
  MATLAB Function : MATLAB Function  TreatAsAtomicUnit=on
  p : Scope
  rollPitchYaw : Scope
  wires:
  "CoM6D ->  CoMXYZ2"/1 -> p/1
  H/1 -> "CoM6D ->  CoMXYZ2"/1, Hom/1, "CoM6D ->  CoMXYZ1"/1
  "CoM6D ->  CoMXYZ1"/1 -> MATLAB Function/1(R)
  MATLAB Function/1(rollPitchYaw) -> rollPitchYaw/1

== system torqueBalancing/DesValues/State Machine/visualise inertial/Visualize hom transf5 ==
  H : Inport
  "CoM6D ->  CoMXYZ1" : Selector  NumberOfDimensions=2  InputPortWidth=7  IndexOptions=Index vector (dialog),Index vector (dialog)  Indices=[1 2 3],[1 2 3]  OutputSizes=1,1
  Hom : Scope
  MATLAB Function : MATLAB Function  TreatAsAtomicUnit=on
  p : Scope
  position : Selector  NumberOfDimensions=2  InputPortWidth=7  IndexOptions=Index vector (dialog),Index vector (dialog)  Indices=[1 2 3],[4]  OutputSizes=1,1
  rollPitchYaw : Scope
  wires:
  position/1 -> p/1  "position"
  H/1 -> position/1, Hom/1, "CoM6D ->  CoMXYZ1"/1  "H"
  "CoM6D ->  CoMXYZ1"/1 -> MATLAB Function/1(R)
  MATLAB Function/1(rollPitchYaw) -> rollPitchYaw/1  "rollPitchYaw"

== system torqueBalancing/DesValues/State Machine/visualise inertial/Visualize hom transf6 ==
  H : Inport
  "CoM6D ->  CoMXYZ1" : Selector  NumberOfDimensions=2  InputPortWidth=7  IndexOptions=Index vector (dialog),Index vector (dialog)  Indices=[1 2 3],[1 2 3]  OutputSizes=1,1
  "CoM6D ->  CoMXYZ2" : Selector  NumberOfDimensions=2  InputPortWidth=7  IndexOptions=Index vector (dialog),Index vector (dialog)  Indices=[1 2 3],[4]  OutputSizes=1,1
  Hom : Scope
  MATLAB Function : MATLAB Function  TreatAsAtomicUnit=on
  p : Scope
  rollPitchYaw : Scope
  wires:
  "CoM6D ->  CoMXYZ2"/1 -> p/1
  H/1 -> "CoM6D ->  CoMXYZ2"/1, Hom/1, "CoM6D ->  CoMXYZ1"/1
  "CoM6D ->  CoMXYZ1"/1 -> MATLAB Function/1(R)
  MATLAB Function/1(rollPitchYaw) -> rollPitchYaw/1

== system torqueBalancing/DesValues/State Machine/visualise inertial/l_sole_H_root_link2 ==
  qj : Inport
  Constant5 : Constant  Value=eye(4)
  Constant6 : Constant  Value=eye(4)
  Inv\* : Product  Inputs=/*  Multiplication=Matrix(*)
  Visualize hom transf4 : Subsystem
  link_name : WBToolboxLibrary/wholeBodyModel/Kinematics/Forward Kinematics  frameName=link_name  robotName=WBT_robotName  localName=WBT_modelName  wbiFile=WBT_wbiFilename  wbiList=WBT_wbiList
  root_link : WBToolboxLibrary/wholeBodyModel/Kinematics/Forward Kinematics  frameName=root_link_name  robotName=WBT_robotName  localName=WBT_modelName  wbiFile=WBT_wbiFilename  wbiList=WBT_wbiList
  link_name_H_root_link : Outport
  wires:
  Constant5/1 -> link_name/1
  Inv\*/1 -> link_name_H_root_link/1  "link_name_H_root_link"
  link_name/1 -> Inv\*/1
  Constant6/1 -> root_link/1
  qj/1 -> link_name/2, root_link/2
  root_link/1 -> Visualize hom transf4/1(H), Inv\*/2

== system torqueBalancing/DesValues/State Machine/visualise inertial/l_sole_H_root_link3 ==
  qj : Inport
  Constant5 : Constant  Value=eye(4)
  Constant6 : Constant  Value=eye(4)
  Inv\* : Product  Inputs=/*  Multiplication=Matrix(*)
  Visualize hom transf4 : Subsystem
  link_name : WBToolboxLibrary/wholeBodyModel/Kinematics/Forward Kinematics  frameName=link_name  robotName=WBT_robotName  localName=WBT_modelName  wbiFile=WBT_wbiFilename  wbiList=WBT_wbiList
  root_link : WBToolboxLibrary/wholeBodyModel/Kinematics/Forward Kinematics  frameName=root_link_name  robotName=WBT_robotName  localName=WBT_modelName  wbiFile=WBT_wbiFilename  wbiList=WBT_wbiList
  link_name_H_root_link : Outport
  wires:
  Constant5/1 -> link_name/1
  Inv\*/1 -> link_name_H_root_link/1  "link_name_H_root_link"
  link_name/1 -> Inv\*/1
  Constant6/1 -> root_link/1
  qj/1 -> link_name/2, root_link/2
  root_link/1 -> Visualize hom transf4/1(H), Inv\*/2

== system torqueBalancing/DesValues/State Machine/visualise inertial/w_H_root_link1 ==
  qj : Inport
  inertial : Inport  Port=2
  "CoM6D ->  CoMXYZ1" : Selector  NumberOfDimensions=2  InputPortWidth=7  IndexOptions=Index vector (dialog),Index vector (dialog)  Indices=[1 2 3],[1 2 3]  OutputSizes=1,1
  Constant : Constant  Value=zeros(3,1)
  Constant2 : Constant  Value=eye(4)
  Constant5 : Constant  Value=eye(4)
  Constant6 : Constant  Value=eye(4)
  Gain : Gain  Gain=pi/180
  Head state : WBToolboxLibrary/Utilities/Yarp Read  portName=[WBT_robotName, '/head/state:o']  signalSize=6  blocking=off  timestamp=off  autoconnect=on  errorOnConnection=off
  Inv\* : Product  Inputs=/*  Multiplication=Matrix(*)
  Inv\*1 : Product  Inputs=/*  Multiplication=Matrix(*)
  Inv\*2 : Product  Inputs=/  Multiplication=Matrix(*)
  Product : Product  Multiplication=Matrix(*)
  Selector : Selector  InputPortWidth=12  IndexOptions=Index vector (dialog)  Indices=[4 5 6 ]  OutputSizes=1
  Selector1 : Selector  InputPortWidth=6  IndexOptions=Index vector (dialog)  Indices=[1:3]  OutputSizes=1
  Switch : Switch  Criteria=u2 > Threshold
  Switch6 : Switch  Criteria=u2 > Threshold
  USE_IMU4EST_BASE : Constant  Value=CONFIG.USE_IMU4EST_BASE
  USE_IMU4EST_BASE1 : Constant  Value=CONFIG.CORRECT_NECK_IMU
  fromImuToHomogeousTransformFCN : MATLAB Function  TreatAsAtomicUnit=on
  holder 1 : WBToolboxLibrary/Utilities/holder 
  holder 2 : WBToolboxLibrary/Utilities/holder 
  imu : WBToolboxLibrary/wholeBodyModel/Kinematics/Forward Kinematics  frameName=imu_link_name  robotName=WBT_robotName  localName=WBT_modelName  wbiFile=WBT_wbiFilename  wbiList=WBT_wbiList
  l_sole_acc : Scope
  link : WBToolboxLibrary/wholeBodyModel/Kinematics/Forward Kinematics  frameName=link_name  robotName=WBT_robotName  localName=WBT_modelName  wbiFile=WBT_wbiFilename  wbiList=WBT_wbiList
  root_link : WBToolboxLibrary/wholeBodyModel/Kinematics/Forward Kinematics  frameName=root_link_name  robotName=WBT_robotName  localName=WBT_modelName  wbiFile=WBT_wbiFilename  wbiList=WBT_wbiList
  w_H_root : Outport
  wires:
  Constant5/1 -> imu/1
  Inv\*/1 -> Inv\*2/1, holder 1/1, fromImuToHomogeousTransformFCN/1(imu_H_link)  "imu_H_link"
  imu/1 -> Inv\*/1
  Constant6/1 -> link/1
  Inv\*1/1 -> Switch6/3, fromImuToHomogeousTransformFCN/3(link_H_root)  "link_H_root"
  link/1 -> Inv\*/2, Inv\*1/1
  inertial/1 -> Selector/1, holder 2/1, fromImuToHomogeousTransformFCN/5(inertial)
  Switch6/1 -> w_H_root/1
  USE_IMU4EST_BASE/1 -> Switch6/2
  fromImuToHomogeousTransformFCN/1(w_H_root) -> Switch6/1
  Constant2/1 -> root_link/1
  qj/1 -> root_link/2, link/2, imu/2
  root_link/1 -> Inv\*1/2
  holder 1/1 -> fromImuToHomogeousTransformFCN/2(imu_H_link_0)
  holder 2/1 -> fromImuToHomogeousTransformFCN/4(inertial_0)
  Inv\*2/1 -> "CoM6D ->  CoMXYZ1"/1
  "CoM6D ->  CoMXYZ1"/1 -> Product/1  "l_sole_R_imu"
  Selector/1 -> Product/2  "imu_acce"
  Product/1 -> l_sole_acc/1
  Head state/1 -> Gain/1
  Selector1/1 -> Switch/1  "neck"
  USE_IMU4EST_BASE1/1 -> Switch/2
  Switch/1 -> fromImuToHomogeousTransformFCN/6(neck)
  Gain/1 -> Selector1/1
  Constant/1 -> Switch/3

== system torqueBalancing/DesValues/State Machine/visualise inertial/w_H_root_link4 ==
  qj : Inport
  inertial : Inport  Port=2
  "CoM6D ->  CoMXYZ1" : Selector  NumberOfDimensions=2  InputPortWidth=7  IndexOptions=Index vector (dialog),Index vector (dialog)  Indices=[1 2 3],[1 2 3]  OutputSizes=1,1
  Constant : Constant  Value=zeros(3,1)
  Constant2 : Constant  Value=eye(4)
  Constant5 : Constant  Value=eye(4)
  Constant6 : Constant  Value=eye(4)
  Gain : Gain  Gain=pi/180
  Head state : WBToolboxLibrary/Utilities/Yarp Read  portName=[WBT_robotName, '/head/state:o']  signalSize=6  blocking=off  timestamp=off  autoconnect=on  errorOnConnection=off
  Inv\* : Product  Inputs=/*  Multiplication=Matrix(*)
  Inv\*1 : Product  Inputs=/*  Multiplication=Matrix(*)
  Inv\*2 : Product  Inputs=/  Multiplication=Matrix(*)
  Product : Product  Multiplication=Matrix(*)
  Selector : Selector  InputPortWidth=12  IndexOptions=Index vector (dialog)  Indices=[4 5 6 ]  OutputSizes=1
  Selector1 : Selector  InputPortWidth=6  IndexOptions=Index vector (dialog)  Indices=[1:3]  OutputSizes=1
  Switch : Switch  Criteria=u2 > Threshold
  Switch6 : Switch  Criteria=u2 > Threshold
  USE_IMU4EST_BASE : Constant  Value=CONFIG.USE_IMU4EST_BASE
  USE_IMU4EST_BASE1 : Constant  Value=CONFIG.CORRECT_NECK_IMU
  fromImuToHomogeousTransformFCN : MATLAB Function  TreatAsAtomicUnit=on
  holder 1 : WBToolboxLibrary/Utilities/holder 
  holder 2 : WBToolboxLibrary/Utilities/holder 
  imu : WBToolboxLibrary/wholeBodyModel/Kinematics/Forward Kinematics  frameName=imu_link_name  robotName=WBT_robotName  localName=WBT_modelName  wbiFile=WBT_wbiFilename  wbiList=WBT_wbiList
  l_sole_acc : Scope
  link : WBToolboxLibrary/wholeBodyModel/Kinematics/Forward Kinematics  frameName=link_name  robotName=WBT_robotName  localName=WBT_modelName  wbiFile=WBT_wbiFilename  wbiList=WBT_wbiList
  root_link : WBToolboxLibrary/wholeBodyModel/Kinematics/Forward Kinematics  frameName=root_link_name  robotName=WBT_robotName  localName=WBT_modelName  wbiFile=WBT_wbiFilename  wbiList=WBT_wbiList
  w_H_root : Outport
  wires:
  Constant5/1 -> imu/1
  Inv\*/1 -> Inv\*2/1, holder 1/1, fromImuToHomogeousTransformFCN/1(imu_H_link)  "imu_H_link"
  imu/1 -> Inv\*/1
  Constant6/1 -> link/1
  Inv\*1/1 -> Switch6/3, fromImuToHomogeousTransformFCN/3(link_H_root)  "link_H_root"
  link/1 -> Inv\*/2, Inv\*1/1
  inertial/1 -> Selector/1, holder 2/1, fromImuToHomogeousTransformFCN/5(inertial)
  Switch6/1 -> w_H_root/1
  USE_IMU4EST_BASE/1 -> Switch6/2
  fromImuToHomogeousTransformFCN/1(w_H_root) -> Switch6/1
  Constant2/1 -> root_link/1
  qj/1 -> root_link/2, link/2, imu/2
  root_link/1 -> Inv\*1/2
  holder 1/1 -> fromImuToHomogeousTransformFCN/2(imu_H_link_0)
  holder 2/1 -> fromImuToHomogeousTransformFCN/4(inertial_0)
  Inv\*2/1 -> "CoM6D ->  CoMXYZ1"/1
  "CoM6D ->  CoMXYZ1"/1 -> Product/1  "l_sole_R_imu"
  Selector/1 -> Product/2  "imu_acce"
  Product/1 -> l_sole_acc/1
  Head state/1 -> Gain/1
  Selector1/1 -> Switch/1  "neck"
  USE_IMU4EST_BASE1/1 -> Switch/2
  Switch/1 -> fromImuToHomogeousTransformFCN/6(neck)
  Gain/1 -> Selector1/1
  Constant/1 -> Switch/3

== system torqueBalancing/DesValues/State Machine/visualise inertial/l_sole_H_root_link2/Visualize hom transf4 ==
  H : Inport
  "CoM6D ->  CoMXYZ1" : Selector  NumberOfDimensions=2  InputPortWidth=7  IndexOptions=Index vector (dialog),Index vector (dialog)  Indices=[1 2 3],[1 2 3]  OutputSizes=1,1
  "CoM6D ->  CoMXYZ2" : Selector  NumberOfDimensions=2  InputPortWidth=7  IndexOptions=Index vector (dialog),Index vector (dialog)  Indices=[1 2 3],[4]  OutputSizes=1,1
  Hom : Scope
  R : Scope
  p : Scope
  wires:
  "CoM6D ->  CoMXYZ1"/1 -> R/1
  "CoM6D ->  CoMXYZ2"/1 -> p/1
  H/1 -> "CoM6D ->  CoMXYZ2"/1, Hom/1, "CoM6D ->  CoMXYZ1"/1

== system torqueBalancing/DesValues/State Machine/visualise inertial/l_sole_H_root_link3/Visualize hom transf4 ==
  H : Inport
  "CoM6D ->  CoMXYZ1" : Selector  NumberOfDimensions=2  InputPortWidth=7  IndexOptions=Index vector (dialog),Index vector (dialog)  Indices=[1 2 3],[1 2 3]  OutputSizes=1,1
  "CoM6D ->  CoMXYZ2" : Selector  NumberOfDimensions=2  InputPortWidth=7  IndexOptions=Index vector (dialog),Index vector (dialog)  Indices=[1 2 3],[4]  OutputSizes=1,1
  Hom : Scope
  R : Scope
  p : Scope
  wires:
  "CoM6D ->  CoMXYZ1"/1 -> R/1
  "CoM6D ->  CoMXYZ2"/1 -> p/1
  H/1 -> "CoM6D ->  CoMXYZ2"/1, Hom/1, "CoM6D ->  CoMXYZ1"/1

== matlab function DesValues/State Machine/visualise inertial/w_H_root_link1/fromImuToHomogeousTransformFCN ==
  data: imu_H_link input double; imu_H_link_0 input double; link_H_root input double; inertial_0 input double; inertial input double; neck input double; w_H_root output double; CONFIG parameter double
function w_H_root = fromBaseToWorldWithImuFCN(imu_H_link,imu_H_link_0,link_H_root,inertial_0,inertial,neck,CONFIG)
%#codegen
w_H_root = fromBaseToWorldWithImu(imu_H_link,imu_H_link_0,link_H_root,inertial_0,inertial,neck,CONFIG);

== matlab function DesValues/Internal coordinator/w_H_root_link4/fromImuToHomogeousTransformFCN ==
  data: imu_H_link input double; imu_H_link_0 input double; link_H_root input double; inertial_0 input double; inertial input double; neck input double; w_H_root output double; CONFIG parameter double
function w_H_root = fromBaseToWorldWithImuFCN(imu_H_link,imu_H_link_0,link_H_root,inertial_0,inertial,neck,CONFIG)
%#codegen
w_H_root = fromBaseToWorldWithImu(imu_H_link,imu_H_link_0,link_H_root,inertial_0,inertial,neck,CONFIG);

== matlab function DesValues/MATLAB Function ==
  data: w_H_b_vectorised input double; w_H_b output double; foot_p_b input double; rollPitchYaw output double
function [w_H_b,rollPitchYaw] = buildHomogenousTranformation(w_H_b_vectorised,foot_p_b)
%#codegen

w_H_b = [w_H_b_vectorised(1:4),w_H_b_vectorised(5:8),w_H_b_vectorised(9:12),...
         w_H_b_vectorised(13:16)];

w_H_b(1:3,4) = foot_p_b;
rollPitchYaw = rollPitchYawFromRotation(w_H_b(1:3,1:3));
rollPitchYaw(3) = 0;

== matlab function DesValues/State Machine Walking/nu/MATLAB Function ==
  data: JcLeftFoot input double; JcRightFoot input double; activeFeetConstraints input double; y output double; qD input double; reg parameter double
function y = fcn(JcLeftFoot,JcRightFoot,activeFeetConstraints,qD,reg)
%#codegen

Jc = [activeFeetConstraints(1)*JcLeftFoot;
      activeFeetConstraints(2)*JcRightFoot];

pinvJb = (Jc(:,1:6)'*Jc(:,1:6) + reg.pinvDampVb*eye(6))\Jc(:,1:6)';  
  
% pinvJb = pinv(Jc(:,1:6));

y = -pinvJb*Jc(:,7:end)*qD;

== matlab function DesValues/State Machine Walking/stateMachineFCN ==
  data: connection input double; wrench_rightFoot input double; wrench_leftFoot input double; CoM_0 input double; q0 input double; w_CoM input double; CoMIn input double; qIn input double; constraintsIn input double; w_H_b output double; CoMDes output double; qDes output double; constraints output double; l_sole_H_b input double; r_sole_H_b input double; sm parameter double; impedances output double; gain parameter double; currentState output double
function [w_H_b, CoMDes,qDes,constraints,impedances,currentState] = ...
    stateMachineFCN(connection,wrench_rightFoot,wrench_leftFoot,CoM_0, q0, w_CoM , CoMIn, qIn, constraintsIn, l_sole_H_b, r_sole_H_b, sm,gain)
%#codegen
 
[CoMDes,qDes,constraints, currentState,impedances,w_H_b] = ...
    stateMachineWalking(connection,CoM_0, q0, w_CoM, CoMIn, qIn, constraintsIn, wrench_rightFoot,wrench_leftFoot,l_sole_H_b, r_sole_H_b, sm,gain);

== matlab function DesValues/Internal coordinator/nu/MATLAB Function ==
  data: JcLeftFoot input double; JcRightFoot input double; activeFeetConstraints input double; y output double; qD input double; reg parameter double
function y = fcn(JcLeftFoot,JcRightFoot,activeFeetConstraints,qD,reg)
%#codegen

Jc = [activeFeetConstraints(1)*JcLeftFoot;
      activeFeetConstraints(2)*JcRightFoot];

pinvJb = (Jc(:,1:6)'*Jc(:,1:6) + reg.pinvDampVb*eye(6))\Jc(:,1:6)';  
  
% pinvJb = pinv(Jc(:,1:6));

y = -pinvJb*Jc(:,7:end)*qD;

== matlab function DesValues/State Machine/w_H_root_link4/fromImuToHomogeousTransformFCN ==
  data: imu_H_link input double; imu_H_link_0 input double; link_H_root input double; inertial_0 input double; inertial input double; neck input double; w_H_root output double; CONFIG parameter double
function w_H_root = fromBaseToWorldWithImuFCN(imu_H_link,imu_H_link_0,link_H_root,inertial_0,inertial,neck,CONFIG)
%#codegen
w_H_root = fromBaseToWorldWithImu(imu_H_link,imu_H_link_0,link_H_root,inertial_0,inertial,neck,CONFIG);

== matlab function DesValues/State Machine/w_H_root_link1/fromImuToHomogeousTransformFCN ==
  data: imu_H_link input double; imu_H_link_0 input double; link_H_root input double; inertial_0 input double; inertial input double; neck input double; w_H_root output double; CONFIG parameter double
function w_H_root = fromBaseToWorldWithImuFCN(imu_H_link,imu_H_link_0,link_H_root,inertial_0,inertial,neck,CONFIG)
%#codegen
w_H_root = fromBaseToWorldWithImu(imu_H_link,imu_H_link_0,link_H_root,inertial_0,inertial,neck,CONFIG);

== matlab function DesValues/Internal coordinator/refGen/refGenFCN ==
  data: xCom0 input double; qDes output double; q0 input double; t input double; references parameter double; desired_x_dx_ddx_CoM output double
function [qDes,desired_x_dx_ddx_CoM] = refGenFCN(xCom0,q0,t,references)
%#codegen

[qDes,desired_x_dx_ddx_CoM] = refGen(xCom0,q0,t,references);

== matlab function DesValues/State Machine Walking/w_H_root_link4/fromImuToHomogeousTransformFCN ==
  data: imu_H_link input double; imu_H_link_0 input double; link_H_root input double; inertial_0 input double; inertial input double; neck input double; w_H_root output double; CONFIG parameter double
function w_H_root = fromBaseToWorldWithImuFCN(imu_H_link,imu_H_link_0,link_H_root,inertial_0,inertial,neck,CONFIG)
%#codegen
w_H_root = fromBaseToWorldWithImu(imu_H_link,imu_H_link_0,link_H_root,inertial_0,inertial,neck,CONFIG);
